simulink model "harness"  (R2021b)
settings: Solver=FixedStepAuto  StartTime=0.0  StopTime=inf  FixedStep=1/1000  RelTol=1e-3
libraries: simulink x1
settings Model: PacingRate=3  Creator=DAUIN-Win10  LastModifiedBy=sagai
settings SolverCC: AllowMultiTaskInputOutput=on  ConcurrentTasks=on  AutoInsertRateTranBlk=on

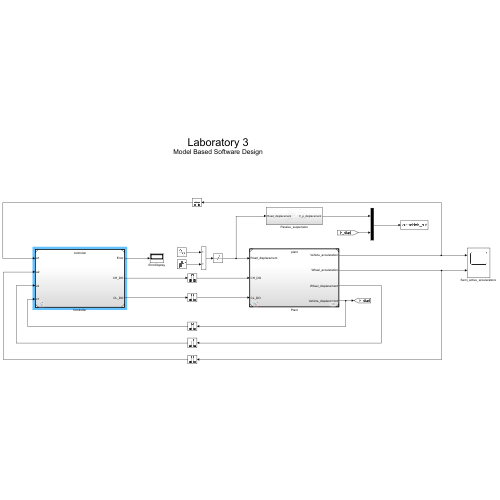
[thumbnail: Simulink's stored preview of the top-level diagram]
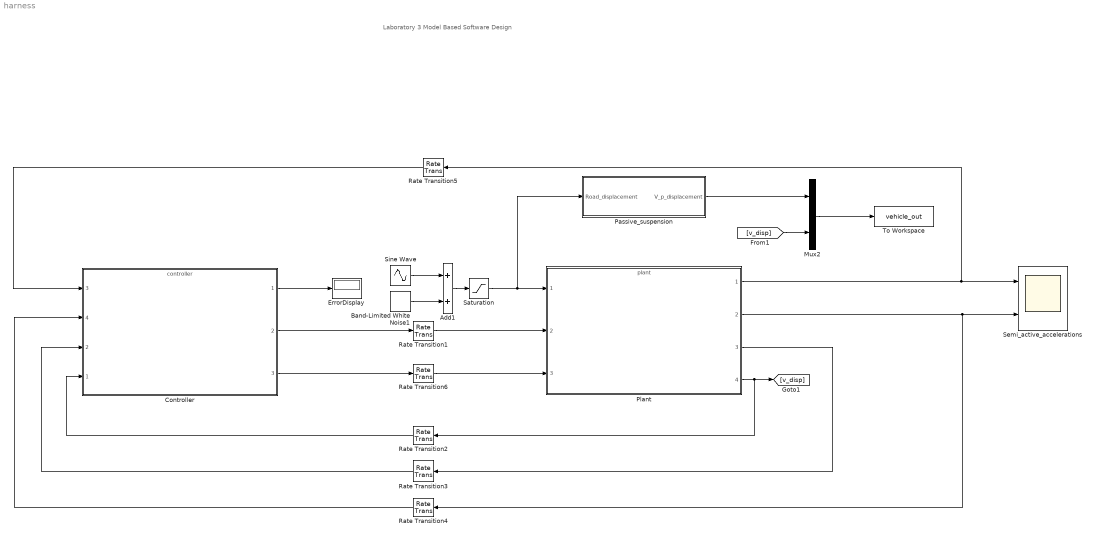
== system harness ==
  note: Laboratory 3
      | Model Based Software Design
  Add1 : Sum
  Band-Limited White Noise1 : simulink/Sources/Band-Limited White Noise  Cov=[0.0000001]  Ts=0.005  seed=[23341]
  Controller : ModelReference  ModelNameDialog=controller  SimulationMode=Normal  ModelReferenceVersion=1.68
      settings: PortSchema="{\"entries\":[{\"content\":{\"sides\":[{\"content\":{\"connectorIds\":[\"In3\",\"In4\",\"In2\",\"In1\"]},\"type\":\"ConnectorPlacement.EquallySpacedRectSide\",\"uuid\":\"5d4bcb7a-15ff-4650-938d-06bf098fb6b9\"},{\"content\":{\"connectorIds\":[\"Out1\",\"Out2\",\"Out3\"],\"side\":\"RIGHT\"},\"type\":\"ConnectorPlacement.EquallySpacedRectSide\",\"uuid\":\"e59f410d-5c8a-489b-98c9-f6a894bced9b\"},{\"content\":{\"connectorIds\":[],\"side\":\"TOP\"},\"type\":\"ConnectorPlacement.EquallySpacedRectSide\",\"uuid\":\"f3e4af64-d7c8-4919-ad88-7d60610a0d24\"}]},\"type\":\"ConnectorPlacement.EquallySpacedConnector\",\"uuid\":\"7927880e-c3da-4df5-9834-46bd773e0ad2\"}],\"packageUris\":[\"http://schema.mathworks.com/mf0/Connector/R2020b\"],\"version\":\"1.0\"}"
  ErrorDisplay : Display
  Mux2 : Mux  Inputs=2
  Passive_suspension : Subsystem
  Plant : ModelReference  ModelNameDialog=plant  SimulationMode=Normal  ModelReferenceVersion=1.17
  Rate Transition{1..6} (6 alike) : RateTransition
  Saturation : Saturate  UpperLimit=0.2  LowerLimit=-0.2
  Semi_active_accelerations : Scope  NumInputPorts=2
  Sine Wave : Sin  Amplitude=0.2  Frequency=3  Phase=0.5  SampleTime=0
  To Workspace : ToWorkspace  VariableName=vehicle_out  SaveFormat=Timeseries  SampleTime=-1
  wires:
  Controller/1 -> ErrorDisplay/1
  Plant/3 -> Rate Transition3/1
  Rate Transition3/1 -> Controller/2
  Rate Transition2/1 -> Controller/1
  Plant/1 -> Semi_active_accelerations/1, Rate Transition5/1
  Controller/2 -> Rate Transition1/1
  Controller/3 -> Rate Transition6/1
  Rate Transition4/1 -> Controller/4
  Rate Transition5/1 -> Controller/3
  Rate Transition1/1 -> Plant/2
  Rate Transition6/1 -> Plant/3
  Plant/2 -> Rate Transition4/1, Semi_active_accelerations/2
  Sine Wave/1 -> Add1/1
  Add1/1 -> Saturation/1
  Band-Limited White Noise1/1 -> Add1/2
  Saturation/1 -> Passive_suspension/1(Road_displacement), Plant/1
  Mux2/1 -> To Workspace/1
  Plant/4 -> [v_disp], Rate Transition2/1
  Passive_suspension/1(V_p_displacement) -> Mux2/1
  [v_disp] -> Mux2/2

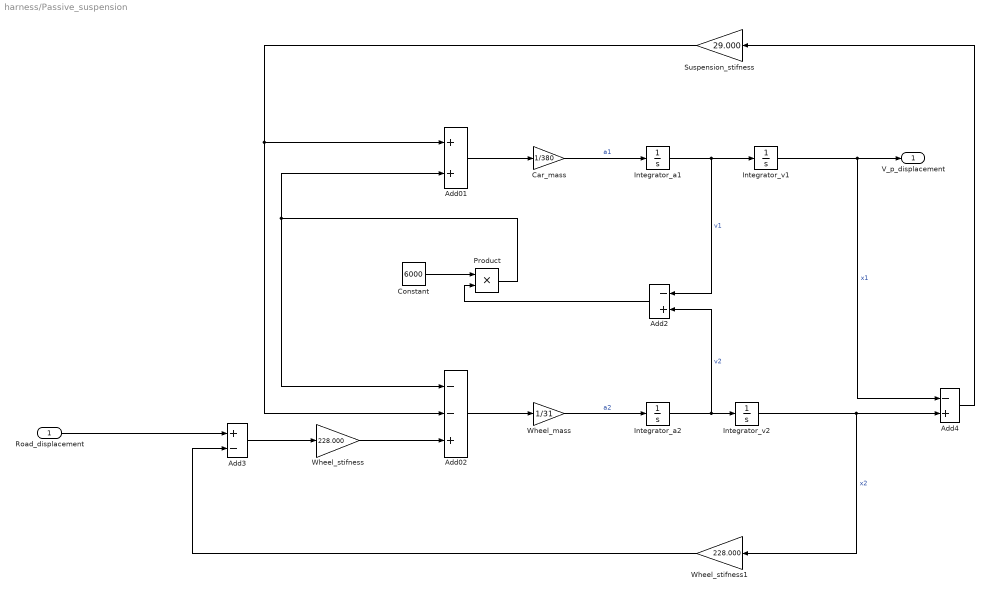
== system harness/Passive_suspension ==
  Road_displacement : Inport
  Add01 : Sum
  Add02 : Sum  Inputs=--+
  Add2 : Sum  Inputs=-+
  Add3 : Sum  Inputs=+-
  Add4 : Sum  Inputs=-+
  Car_mass : Gain  Gain=1/380
  Constant : Constant  Value=6000
  Integrator_a1 : Integrator
  Integrator_a2 : Integrator
  Integrator_v1 : Integrator
  Integrator_v2 : Integrator
  Product : Product
  Suspension_stifness : Gain  Gain=29.000
  Wheel_mass : Gain  Gain=1/31
  Wheel_stifness : Gain  Gain=228.000
  Wheel_stifness1 : Gain  Gain=228.000
  V_p_displacement : Outport
  wires:
  Road_displacement/1 -> Add3/1
  Car_mass/1 -> Integrator_a1/1  "a1"
  Add02/1 -> Wheel_mass/1
  Wheel_stifness1/1 -> Add3/2
  Product/1 -> Add01/2, Add02/1
  Add01/1 -> Car_mass/1
  Add3/1 -> Wheel_stifness/1
  Add4/1 -> Suspension_stifness/1
  Integrator_a2/1 -> Add2/2, Integrator_v2/1  "v2"
  Integrator_a1/1 -> Add2/1, Integrator_v1/1  "v1"
  Constant/1 -> Product/1
  Add2/1 -> Product/2
  Suspension_stifness/1 -> Add01/1, Add02/2
  Integrator_v1/1 -> V_p_displacement/1, Add4/1  "x1"
  Wheel_stifness/1 -> Add02/3
  Integrator_v2/1 -> Add4/2, Wheel_stifness1/1  "x2"
  Wheel_mass/1 -> Integrator_a2/1  "a2"
